simulink model "Colas_con_varios_servidores"  (R2023a)
settings: Solver=VariableStepAuto  StartTime=0.0  StopTime=10.0  RelTol=1e-3
undefined symbols (not defined in the file): m
settings Model: Creator=santi  LastModifiedBy=santi

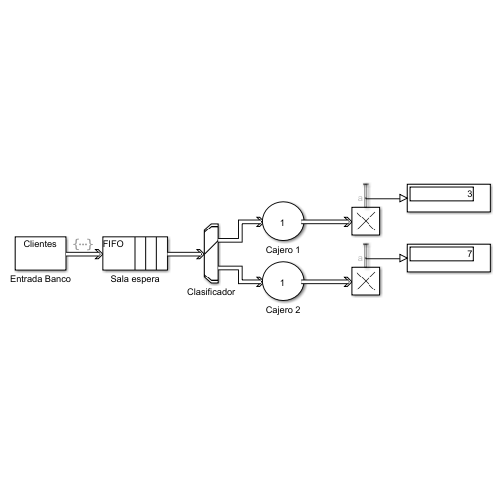
[thumbnail: Simulink's stored preview of the top-level diagram]
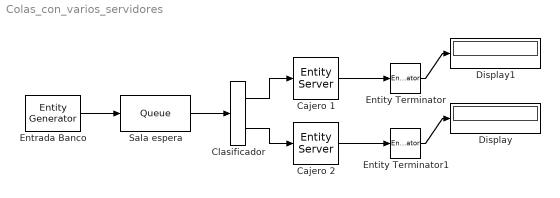
== system Colas_con_varios_servidores ==
  Cajero 1 : EntityServer  InputPortMessageModes=m  OutputPortMessageModes=m  Capacity=1
  Cajero 2 : EntityServer  InputPortMessageModes=m  OutputPortMessageModes=m  Capacity=1
  Clasificador : EntityOutputSwitch  InputPortMessageModes=m  OutputPortMessageModes=m,m  SwitchingCriterion=From attribute  SwitchAttributeName=TransaccionTipo
  Display : Display
  Display1 : Display
  Entity Terminator : EntityTerminator  InputPortMessageModes=m  NumberEntitiesArrived=on
      settings: OutputPortMap=o0
  Entity Terminator1 : EntityTerminator  InputPortMessageModes=m  NumberEntitiesArrived=on
      settings: OutputPortMap=o0
  Entrada Banco : EntityGenerator  OutputPortMessageModes=m  AttributeName=TransaccionTipo  AttributeInitialValue=0  EntityType=Structured  EntityTypeName=Clientes
  Sala espera : Queue  InputPortMessageModes=m  OutputPortMessageModes=m  EntryAction=entity.TransaccionTipo = randi([1 2]);
  wires:
  Entrada Banco/1 -> Sala espera/1
  Sala espera/1 -> Clasificador/1
  Clasificador/1 -> Cajero 1/1
  Clasificador/2 -> Cajero 2/1
  Cajero 1/1 -> Entity Terminator/1
  Cajero 2/1 -> Entity Terminator1/1
  Entity Terminator1/1 -> Display/1
  Entity Terminator/1 -> Display1/1
